simulink model "a1_stairs"  (R2022b)
settings: Solver=VariableStepAuto  StartTime=0.0  StopTime=5  FixedStep=0.001  MaxStep=Auto  MinStep=Auto  RelTol=1e-3
values from neighbouring files (symbols this model uses):
  Astate = [A1; A2; A3; A4; A5; A6]    [AME556_HW4_Cornwell.m]    (also in AME_556_Final_Project.m)
  calfd = -1.6    [AME556_HW3_Cornwell.m]    (also in AME_556_Final_Project.m)
  dt = params.dt    [AME556_HW4_Cornwell.m]    (also in AME_556_Final_Project.m = 0.03)
  gait_type = 1    [AME_556_Final_Project.m]
  H = H3    [AME556_HW1_Cornwell.m]    (also in AME556_HW4_Cornwell.m = blkdiag(H,Rmpc); AME_556_Final_Project.m = blkdiag(H,Rmpc))
  hipd = 0    [AME556_HW3_Cornwell.m]    (also in AME_556_Final_Project.m)
  kd = params.kd    [AME556_HW3_Cornwell.m]    (also in AME_556_Final_Project.m = 4)
  kp = params.kp    [AME556_HW3_Cornwell.m]    (also in AME_556_Final_Project.m = 25)
  m = params.m    [AME556_HW3_Cornwell.m]    (also in AME556_HW4_Cornwell.m = params.mass)
  N = size(x, 2)    [AME556_HW3_Cornwell.m]    (also in AME556_HW4_Cornwell.m; AME_556_Final_Project.m = 10)
  PD = 0    [AME_556_Final_Project.m]
  Q = diag([40 50 60 10 10 10 4 4 4 1 1 1 0])    [AME556_HW4_Cornwell.m]    (also in AME_556_Final_Project.m = diag([0 800 15000 49500 14000 5000 1900 700 700 900 700 200 )
  speed = 0.37    [AME_556_Final_Project.m]
  thighd = 0.95    [AME556_HW3_Cornwell.m]    (also in AME_556_Final_Project.m)
  Tstance = 0.15    [AME_556_Final_Project.m]
  X = quadprog(H,f,Astate,bstate,Aeq,beq)    [AME556_HW4_Cornwell.m]
  z0 = [x0(1)-1; x0(2)]    [AME556_HW5_Cornwell.m]    (also in AME_556_Final_Project.m = 0.2855)
  zd = 0.31    [AME_556_Final_Project.m]
undefined symbols (not defined in the file or in its folder): Y, Z
libraries: sm_lib x211, nesl_utility x96
(part 1 of 6)
settings Model: SimulationMode=accelerator  Creator=taracornwell  LastModifiedBy=taracornwell
settings SolverCC: InitialStep=Auto

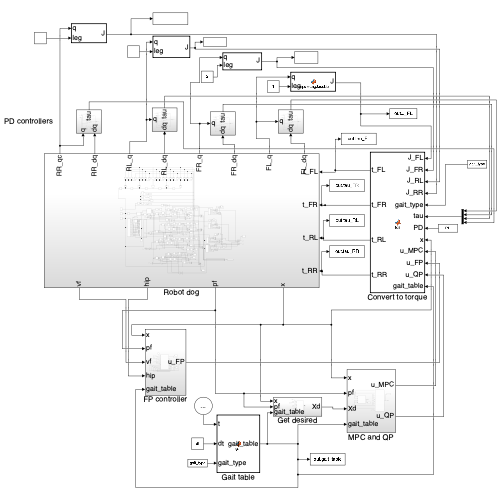
[thumbnail: Simulink's stored preview of the top-level diagram]
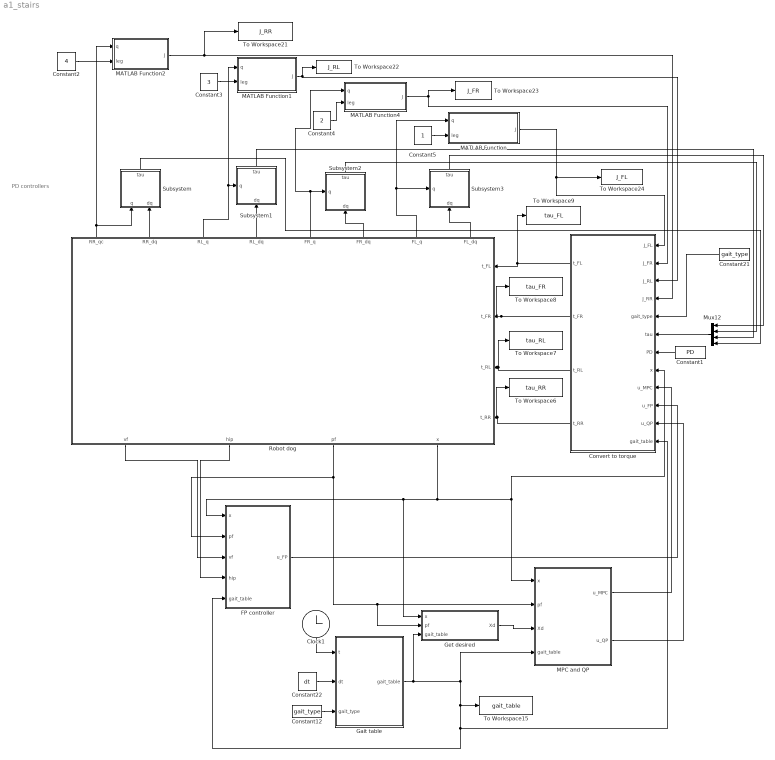
== system a1_stairs ==
  note: PD controllers
  Clock1 : Clock
  Constant1 : Constant  Value=PD
  Constant12 : Constant  Value=gait_type
  Constant2 : Constant  Value=4
  Constant21 : Constant  Value=gait_type
  Constant22 : Constant  Value=dt
  Constant3 : Constant  Value=3
  Constant4 : Constant  Value=2
  Constant5 : Constant
  Convert to torque : MATLAB Function  TreatAsAtomicUnit=on
  FP controller : Subsystem
  Gait table : MATLAB Function  TreatAsAtomicUnit=on
  Get desired : Subsystem
  MATLAB Function : MATLAB Function  TreatAsAtomicUnit=on
  MATLAB Function1 : MATLAB Function  TreatAsAtomicUnit=on
  MATLAB Function2 : MATLAB Function  TreatAsAtomicUnit=on
  MATLAB Function4 : MATLAB Function  TreatAsAtomicUnit=on
  MPC and QP : Subsystem
  Mux12 : Mux
  Robot dog : Subsystem
      settings: PortSchema="{\"entries\":[{\"content\":{\"sides\":[{\"content\":{\"connectorIds\":[]},\"type\":\"ConnectorPlacement.EquallySpacedRectSide\",\"uuid\":\"4b575dd2-8d54-403b-9bc5-5266adaf2c55\"},{\"content\":{\"connectorIds\":[\"In1\",\"In2\",\"In3\",\"In4\"],\"side\":\"RIGHT\"},\"type\":\"ConnectorPlacement.EquallySpacedRectSide\",\"uuid\":\"82527a3b-f9d7-4a8b-bd5e-4f6548b7e261\"},{\"content\":{\"connectorIds\":[\"Out5\",\"Out6\",\"Out7\",\"Out8\",\"Out9\",\"Out10\",\"Out11\",\"Out12\"],\"side\":\"TOP\"},\"type\":\"ConnectorPlacement.EquallySpacedRectSide\",\"uuid\":\"6cf7ade0-7bce-44f1-bdf8-f3f43d85f41e\"},{\"content\":{\"connectorIds\":[\"Out1\",\"Out2\",\"Out3\",\"Out4\"],\"side\":\"BOTTOM\"},\"type\":\"ConnectorPlacement.EquallySpacedRectSide\",\"uuid\":\"259fbb5c-5e02-4470-9968-a6164b709c29\"}]},\"type\":\"ConnectorPlacement.EquallySpacedConnector\",\"uuid\":\"e6132217-986e-4687-b6cf-81846310c900\"}],\"packageUris\":[\"http://schema.mathworks.com/mf0/Connector/R2020b\"],\"version\":\"1.0\"}"
  Subsystem : Subsystem
  Subsystem1 : Subsystem
      settings: PortSchema="{\"entries\":[{\"content\":{\"sides\":[{\"content\":{\"connectorIds\":[\"In1\"]},\"type\":\"ConnectorPlacement.EquallySpacedRectSide\",\"uuid\":\"94da9161-92be-4aef-baf4-8a5634d52659\"},{\"content\":{\"connectorIds\":[\"Out1\"],\"side\":\"RIGHT\"},\"type\":\"ConnectorPlacement.EquallySpacedRectSide\",\"uuid\":\"102a03b1-c4cf-48a2-963b-aa3bfb735113\"},{\"content\":{\"connectorIds\":[\"In2\"],\"side\":\"TOP\"},\"type\":\"ConnectorPlacement.EquallySpacedRectSide\",\"uuid\":\"a02a1465-badb-4128-b0b1-6698ff9b6cc1\"}]},\"type\":\"ConnectorPlacement.EquallySpacedConnector\",\"uuid\":\"0057a81d-01ff-46f4-b9dc-e6ef6b1b9d02\"}],\"packageUris\":[\"http://schema.mathworks.com/mf0/Connector/R2020b\"],\"version\":\"1.0\"}"
  Subsystem2 : Subsystem
      settings: PortSchema="{\"entries\":[{\"content\":{\"sides\":[{\"content\":{\"connectorIds\":[\"In1\"]},\"type\":\"ConnectorPlacement.EquallySpacedRectSide\",\"uuid\":\"94da9161-92be-4aef-baf4-8a5634d52659\"},{\"content\":{\"connectorIds\":[\"Out1\"],\"side\":\"RIGHT\"},\"type\":\"ConnectorPlacement.EquallySpacedRectSide\",\"uuid\":\"102a03b1-c4cf-48a2-963b-aa3bfb735113\"},{\"content\":{\"connectorIds\":[\"In2\"],\"side\":\"TOP\"},\"type\":\"ConnectorPlacement.EquallySpacedRectSide\",\"uuid\":\"a02a1465-badb-4128-b0b1-6698ff9b6cc1\"}]},\"type\":\"ConnectorPlacement.EquallySpacedConnector\",\"uuid\":\"0057a81d-01ff-46f4-b9dc-e6ef6b1b9d02\"}],\"packageUris\":[\"http://schema.mathworks.com/mf0/Connector/R2020b\"],\"version\":\"1.0\"}"
  Subsystem3 : Subsystem
      settings: PortSchema="{\"entries\":[{\"content\":{\"sides\":[{\"content\":{\"connectorIds\":[\"In1\"]},\"type\":\"ConnectorPlacement.EquallySpacedRectSide\",\"uuid\":\"94da9161-92be-4aef-baf4-8a5634d52659\"},{\"content\":{\"connectorIds\":[\"Out1\"],\"side\":\"RIGHT\"},\"type\":\"ConnectorPlacement.EquallySpacedRectSide\",\"uuid\":\"102a03b1-c4cf-48a2-963b-aa3bfb735113\"},{\"content\":{\"connectorIds\":[\"In2\"],\"side\":\"TOP\"},\"type\":\"ConnectorPlacement.EquallySpacedRectSide\",\"uuid\":\"a02a1465-badb-4128-b0b1-6698ff9b6cc1\"}]},\"type\":\"ConnectorPlacement.EquallySpacedConnector\",\"uuid\":\"0057a81d-01ff-46f4-b9dc-e6ef6b1b9d02\"}],\"packageUris\":[\"http://schema.mathworks.com/mf0/Connector/R2020b\"],\"version\":\"1.0\"}"
  To Workspace15 : ToWorkspace  VariableName=gait_table  SampleTime=-1
  To Workspace21 : ToWorkspace  VariableName=J_RR  SampleTime=-1
  To Workspace22 : ToWorkspace  VariableName=J_RL  SampleTime=-1
  To Workspace23 : ToWorkspace  VariableName=J_FR  SampleTime=-1
  To Workspace24 : ToWorkspace  VariableName=J_FL  SampleTime=-1
  To Workspace6 : ToWorkspace  VariableName=tau_RR  SampleTime=-1
  To Workspace7 : ToWorkspace  VariableName=tau_RL  SampleTime=-1
  To Workspace8 : ToWorkspace  VariableName=tau_FR  SampleTime=-1
  To Workspace9 : ToWorkspace  VariableName=tau_FL  SampleTime=-1
  wires:
  Robot dog/11(FL_q) -> Subsystem3/2(q), MATLAB Function/1(q)
  Robot dog/9(FR_q) -> Subsystem2/2(q), MATLAB Function4/1(q)
  Robot dog/7(RL_q) -> Subsystem1/2(q), MATLAB Function1/1(q)
  Robot dog/5(RR_qc) -> Subsystem/1(q), MATLAB Function2/1(q)
  Constant2/1 -> MATLAB Function2/2(leg)
  Constant3/1 -> MATLAB Function1/2(leg)
  Constant4/1 -> MATLAB Function4/2(leg)
  Constant5/1 -> MATLAB Function/2(leg)
  MATLAB Function/1(J) -> Convert to torque/1(J_FL), To Workspace24/1
  MATLAB Function4/1(J) -> Convert to torque/2(J_FR), To Workspace23/1
  MATLAB Function1/1(J) -> Convert to torque/3(J_RL), To Workspace22/1
  MATLAB Function2/1(J) -> To Workspace21/1, Convert to torque/4(J_RR)
  Gait table/1(gait_table) -> FP controller/5(gait_table), Convert to torque/12(gait_table), To Workspace15/1, MPC and QP/4(gait_table), Get desired/3(gait_table)
  Robot dog/4(x) -> FP controller/1(x), Get desired/1(x), MPC and QP/1(x), Convert to torque/8(x)
  Convert to torque/1(t_FL) -> Robot dog/1(t_FL), To Workspace9/1
  Convert to torque/2(t_FR) -> To Workspace8/1, Robot dog/2(t_FR)
  Convert to torque/3(t_RL) -> To Workspace7/1, Robot dog/3(t_RL)
  Convert to torque/4(t_RR) -> To Workspace6/1, Robot dog/4(t_RR)
  Clock1/1 -> Gait table/1(t)
  Constant12/1 -> Gait table/3(gait_type)
  Constant21/1 -> Convert to torque/5(gait_type)
  Constant22/1 -> Gait table/2(dt)
  MPC and QP/1(u_MPC) -> Convert to torque/9(u_MPC)
  MPC and QP/2(u_QP) -> Convert to torque/11(u_QP)
  FP controller/1(u_FP) -> Convert to torque/10(u_FP)
  Robot dog/3(pf) -> Get desired/2(pf), MPC and QP/2(pf), FP controller/2(pf)
  Robot dog/2(hip) -> FP controller/4(hip)
  Robot dog/1(vf) -> FP controller/3(vf)
  Get desired/1(Xd) -> MPC and QP/3(Xd)
  Robot dog/6(RR_dq) -> Subsystem/2(dq)
  Robot dog/8(RL_dq) -> Subsystem1/1(dq)
  Robot dog/10(FR_dq) -> Subsystem2/1(dq)
  Robot dog/12(FL_dq) -> Subsystem3/1(dq)
  Mux12/1 -> Convert to torque/6(tau)
  Subsystem3/1(tau) -> Mux12/1
  Subsystem2/1(tau) -> Mux12/2
  Subsystem1/1(tau) -> Mux12/3
  Subsystem/1(tau) -> Mux12/4
  Constant1/1 -> Convert to torque/7(PD)

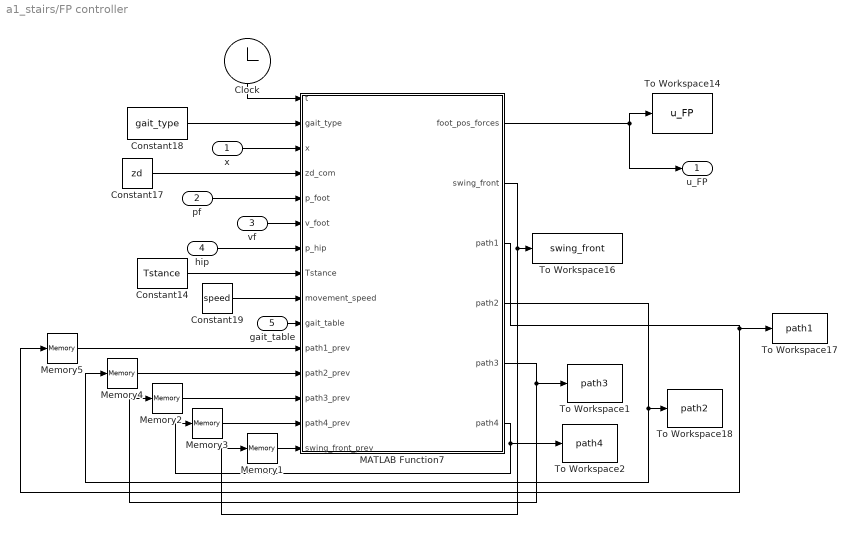
== system a1_stairs/FP controller ==
  x : Inport
  pf : Inport  Port=2
  vf : Inport  Port=3
  hip : Inport  Port=4
  gait_table : Inport  Port=5
  Clock : Clock
  Constant14 : Constant  Value=Tstance
  Constant17 : Constant  Value=zd
  Constant18 : Constant  Value=gait_type
  Constant19 : Constant  Value=speed
  MATLAB Function7 : MATLAB Function  TreatAsAtomicUnit=on
  Memory1 : Memory  InitialCondition=10  InheritSampleTime=on
  Memory{2..5} (4 alike) : Memory  InheritSampleTime=on
  To Workspace1 : ToWorkspace  VariableName=path3  SampleTime=-1
  To Workspace14 : ToWorkspace  VariableName=u_FP  SampleTime=-1
  To Workspace16 : ToWorkspace  VariableName=swing_front  SampleTime=-1
  To Workspace17 : ToWorkspace  VariableName=path1  SampleTime=-1
  To Workspace18 : ToWorkspace  VariableName=path2  SampleTime=-1
  To Workspace2 : ToWorkspace  VariableName=path4  SampleTime=-1
  u_FP : Outport
  wires:
  Constant18/1 -> MATLAB Function7/2(gait_type)
  MATLAB Function7/3(path1) -> To Workspace17/1, Memory5/1
  Clock/1 -> MATLAB Function7/1(t)
  MATLAB Function7/4(path2) -> Memory4/1, To Workspace18/1
  MATLAB Function7/2(swing_front) -> Memory1/1, To Workspace16/1
  Memory5/1 -> MATLAB Function7/11(path1_prev)
  Constant14/1 -> MATLAB Function7/8(Tstance)
  Constant17/1 -> MATLAB Function7/4(zd_com)
  Memory4/1 -> MATLAB Function7/12(path2_prev)
  Constant19/1 -> MATLAB Function7/9(movement_speed)
  MATLAB Function7/1(foot_pos_forces) -> u_FP/1, To Workspace14/1
  x/1 -> MATLAB Function7/3(x)
  pf/1 -> MATLAB Function7/5(p_foot)
  vf/1 -> MATLAB Function7/6(v_foot)
  hip/1 -> MATLAB Function7/7(p_hip)
  gait_table/1 -> MATLAB Function7/10(gait_table)
  Memory1/1 -> MATLAB Function7/15(swing_front_prev)
  Memory2/1 -> MATLAB Function7/13(path3_prev)
  MATLAB Function7/5(path3) -> To Workspace1/1, Memory2/1
  Memory3/1 -> MATLAB Function7/14(path4_prev)
  MATLAB Function7/6(path4) -> To Workspace2/1, Memory3/1

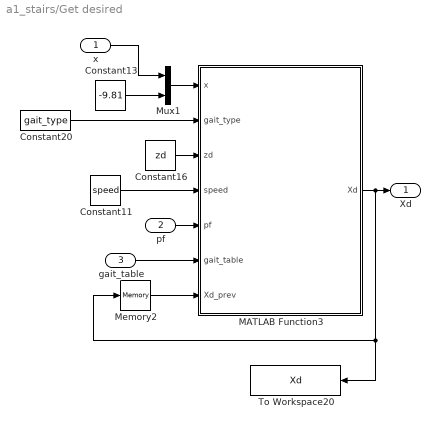
== system a1_stairs/Get desired ==
  x : Inport
  pf : Inport  Port=2
  gait_table : Inport  Port=3
  Constant11 : Constant  Value=speed
  Constant13 : Constant  Value=-9.81
  Constant16 : Constant  Value=zd
  Constant20 : Constant  Value=gait_type
  MATLAB Function3 : MATLAB Function  TreatAsAtomicUnit=on
  Memory2 : Memory  InitialCondition=zeros(13,1)  InheritSampleTime=on
  Mux1 : Mux  Inputs=2
  To Workspace20 : ToWorkspace  VariableName=Xd  SampleTime=-1
  Xd : Outport
  wires:
  pf/1 -> MATLAB Function3/5(pf)
  Mux1/1 -> MATLAB Function3/1(x)
  Constant20/1 -> MATLAB Function3/2(gait_type)
  Constant11/1 -> MATLAB Function3/4(speed)
  Constant13/1 -> Mux1/2
  Constant16/1 -> MATLAB Function3/3(zd)
  MATLAB Function3/1(Xd) -> Memory2/1, To Workspace20/1, Xd/1
  x/1 -> Mux1/1
  Memory2/1 -> MATLAB Function3/7(Xd_prev)
  gait_table/1 -> MATLAB Function3/6(gait_table)

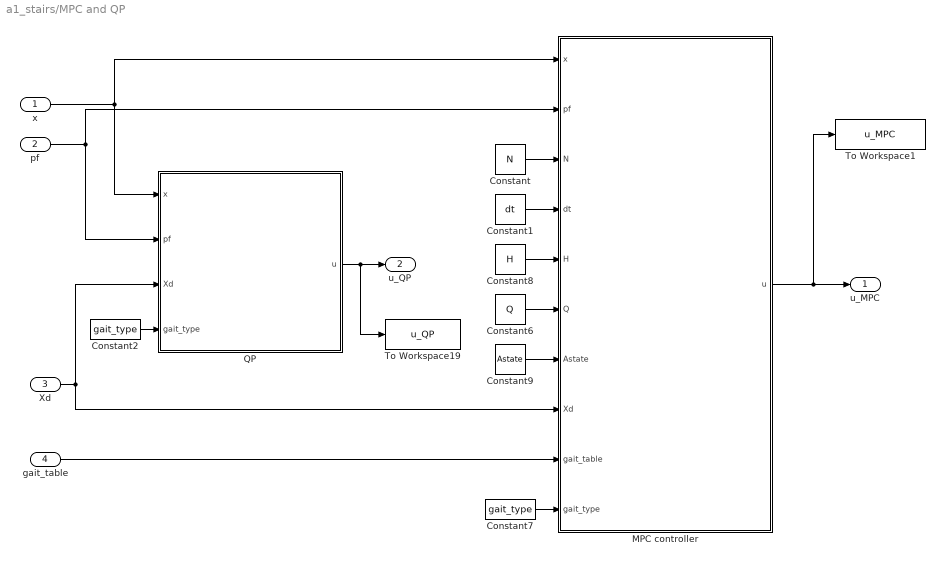
== system a1_stairs/MPC and QP ==
  x : Inport
  pf : Inport  Port=2
  Xd : Inport  Port=3
  gait_table : Inport  Port=4
  Constant : Constant  Value=N
  Constant1 : Constant  Value=dt
  Constant2 : Constant  Value=gait_type
  Constant6 : Constant  Value=Q
  Constant7 : Constant  Value=gait_type
  Constant8 : Constant  Value=H
  Constant9 : Constant  Value=Astate
  MPC controller : MATLAB Function  TreatAsAtomicUnit=on
  "QP " : MATLAB Function  TreatAsAtomicUnit=on
  To Workspace1 : ToWorkspace  VariableName=u_MPC  SampleTime=-1
  To Workspace19 : ToWorkspace  VariableName=u_QP  SampleTime=-1
  u_MPC : Outport
  u_QP : Outport  Port=2
  wires:
  Constant1/1 -> MPC controller/4(dt)
  Constant8/1 -> MPC controller/5(H)
  Constant9/1 -> MPC controller/7(Astate)
  Constant6/1 -> MPC controller/6(Q)
  Constant/1 -> MPC controller/3(N)
  Constant7/1 -> MPC controller/10(gait_type)
  MPC controller/1(u) -> To Workspace1/1, u_MPC/1
  x/1 -> "QP "/1(x), MPC controller/1(x)
  pf/1 -> "QP "/2(pf), MPC controller/2(pf)
  Xd/1 -> "QP "/3(Xd), MPC controller/8(Xd)
  gait_table/1 -> MPC controller/9(gait_table)
  Constant2/1 -> "QP "/4(gait_type)
  "QP "/1(u) -> To Workspace19/1, u_QP/1
